simulink model "AlmostFinishedObserverBlock"  (R2019b)
settings: Solver=VariableStepAuto  StartTime=0.0  StopTime=10.0  RelTol=1e-3
undefined symbols (not defined in the file): M, RTransposed
settings Model: Creator=simen  LastModifiedBy=simen

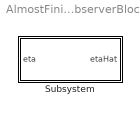
== system AlmostFinishedObserverBlock ==
  Subsystem : Subsystem

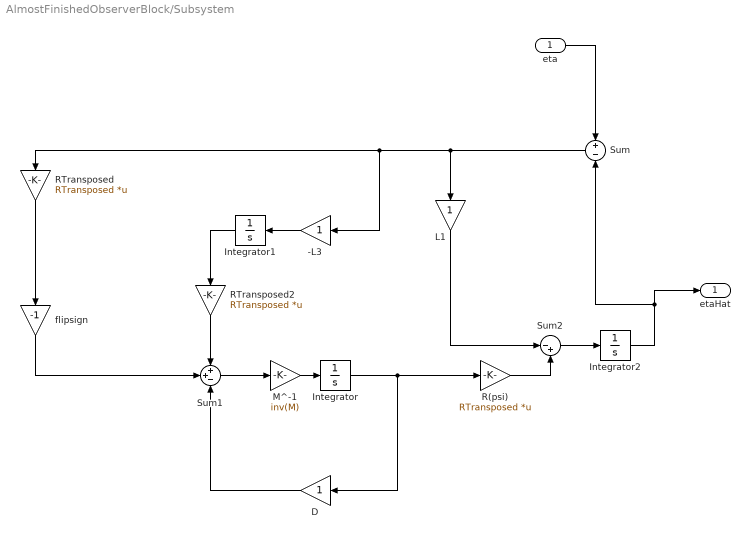
== system AlmostFinishedObserverBlock/Subsystem ==
  eta : Inport
  -L3 : Gain
  D : Gain
  Integrator : Integrator
  Integrator1 : Integrator
  Integrator2 : Integrator
  L1 : Gain
  M^-1 : Gain  Gain=inv(M)
  R(psi) : Gain  Gain=RTransposed  Multiplication=Matrix(K*u)
  RTransposed : Gain  Gain=RTransposed  Multiplication=Matrix(K*u)
  RTransposed2 : Gain  Gain=RTransposed  Multiplication=Matrix(K*u)
  Sum : Sum  Inputs=+|-
  Sum1 : Sum  Inputs=++-
  Sum2 : Sum  Inputs=|-+
  flipsign : Gain  Gain=-1
  etaHat : Outport
  wires:
  Sum/1 -> L1/1, -L3/1, RTransposed/1
  eta/1 -> Sum/1
  RTransposed/1 -> flipsign/1
  M^-1/1 -> Integrator/1
  flipsign/1 -> Sum1/2
  Sum1/1 -> M^-1/1
  D/1 -> Sum1/3
  RTransposed2/1 -> Sum1/1
  Integrator1/1 -> RTransposed2/1
  -L3/1 -> Integrator1/1
  Integrator/1 -> R(psi)/1, D/1
  R(psi)/1 -> Sum2/2
  L1/1 -> Sum2/1
  Sum2/1 -> Integrator2/1
  Integrator2/1 -> etaHat/1, Sum/2
